simulink model "Sample155"  (Simulink 6.3)
settings: Solver=ode45  StartTime=0.0  StopTime=10.0  RelTol=1e-3
libraries: commblkcod2 x1, commrandsrc2 x1, dspbuff3 x1, commdigbbndfm2 x1, commdigbbndcpm2 x1
settings Model: LastModifiedBy=Administrator

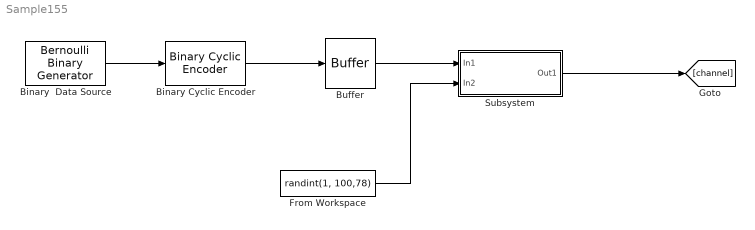
== system Sample155 ==
  Binary Cyclic Encoder : commblkcod2/Binary Cyclic Encoder  n=15  p=[1 1 0 1 0 1]
  Binary  Data Source : commrandsrc2/Bernoulli Binary Generator  P=[0.5]  seed=[12345]  Ts=1.5e-6  frameBased=on  sampPerFrame=10  orient=off  outDataType=double
  Buffer : dspbuff3/Buffer  N=625  V=0  ic=0
  From Workspace : FromWorkspace  VariableName=randint(1, 100,78)  SampleTime=1/1600
  Subsystem : Subsystem
  wires:
  Binary  Data Source/1 -> Binary Cyclic Encoder/1
  Binary Cyclic Encoder/1 -> Buffer/1
  Buffer/1 -> Subsystem/1(In1)
  Subsystem/1(Out1) -> [channel]
  From Workspace/1 -> Subsystem/2(In2)

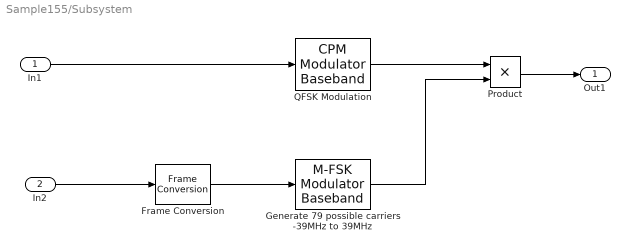
== system Sample155/Subsystem ==
  In1 : Inport
  In2 : Inport  Port=2
  Frame Conversion : FrameConversion
  Generate 79 possible carriers -39MHz to 39MHz : commdigbbndfm2/M-FSK Modulator Baseband  M=79  InType=Integer  Enc=Binary  freqSep=1e6  phaseType=Continuous  numSamp=6.25e4  outDataType=double
  Product : Product  RndMeth=Zero
  QFSK Modulation : commdigbbndcpm2/CPM Modulator Baseband  Mnum=2  inputType=Bit  mappingType=Binary  modIdx=0.3  pulseShape=Gaussian  BT=0.5  mainLobePulseLength=1  rollOff=0.2  pulseLength=1  preHistory=1  phaseOffset=0  samplesPerSymbol=8  outDataType=double
  Out1 : Outport
  wires:
  Product/1 -> Out1/1
  Generate 79 possible carriers -39MHz to 39MHz/1 -> Product/2
  QFSK Modulation/1 -> Product/1
  In1/1 -> QFSK Modulation/1
  Frame Conversion/1 -> Generate 79 possible carriers -39MHz to 39MHz/1
  In2/1 -> Frame Conversion/1
